simulink model "station_no_recovery"  (R2015a)
settings: Solver=ode45  StartTime=0  StopTime=5000  FixedStep=10  MaxStep=1  RelTol=1e-3
(part 1 of 4)
settings Model: Creator=Tzimisce  LastModifiedBy=Tzimisce
settings DebuggingCC: AlgebraicLoopMsg=none  ArtificialAlgebraicLoopMsg=none  InheritedTsInSrcMsg=none

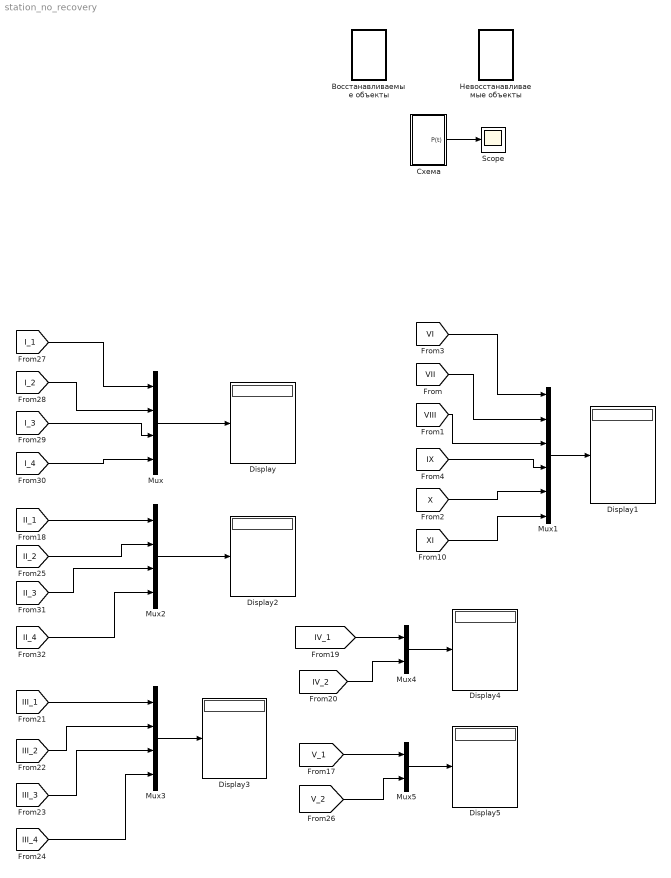
== system station_no_recovery ==
  Display{,1..5} (6 alike) : Display
  Mux : Mux
  Mux1 : Mux  Inputs=6
  Mux2 : Mux
  Mux3 : Mux
  Mux4 : Mux  Inputs=2
  Mux5 : Mux  Inputs=2
  Scope : Scope
      settings: TimeRange=5000
  Восстанавливаемые объекты : Subsystem  mask{lambda_exp1=0.0008664, lambda_norm1=100, M1=800, dp1=0.005, trec_1=5000, Pz1=0, dt1=10000, t_start1_1=0, t_start1_2=50, t_start1_3=100, t_start1_4=200, lambda_exp2=0.0002888, lambda_norm2=300, M2=2400, dp2=0.005, Pz2=0, dt2=10000, t_start2_1=50, t_start2_2=120, t_start2_3=310, t_start2_4=200, lambda_exp3=0.0002888, M3=2400, lambda_norm3=300, dp3=0.005, Pz3=0, dt3=10000, t_start3_1=50, t_start3_2=300, t_start3_3=1000, t_start3_4=150, lambda_exp4=0.0001733, lambda_norm4=500, M4=4000, dp4=0.005, Pz4=0, dt4=10000, t_start4_1=20, t_start4_2=220, lambda_exp5=0.0001733, lambda_norm5=500, M5=4000, dp5=0.005, Pz5=0, dt5=10000, t_start5_1=0, t_start5_2=500, trec_2=8000}
      mask prompts: lambda_exp1 "Параметр экспоненциального распределения ПАЭС"; lambda_norm1 "Параметр нормального распределения ПАЭС"; M1 "Мат ожидание нормального распределения ПАЭС"; dp1 "Доля деградации объекта ПАЭС"; trec_1 "Время капитального ремонта 1"; Pz1 "Заданная вероятность ПАЭС"; dt1 "Время восстановления ПАЭС"; t_start1_1 "Начальная наработка ПАЭС 1"; t_start1_2 "Начальная наработка ПАЭС 2"; t_start1_3 "Начальная наработка ПАЭС 3"; t_start1_4 "Начальная наработка ПАЭС 4"; lambda_exp2 "Параметр экспоненциального распределения УРАЛ"; lambda_norm2 "Параметр нормального распределения УРАЛ"; M2 "Мат ожидание нормального распределения УРАЛ"; dp2 "Доля деградации объекта УРАЛ"; Pz2 "Заданная вероятность УРАЛ"; dt2 "Время восстановления УРАЛ"; t_start2_1 "Начальная наработка УРАЛ 1"; t_start2_2 "Начальная наработка УРАЛ 2"; t_start2_3 "Начальная наработка УРАЛ 3"; t_start2_4 "Начальная наработка УРАЛ 4"; lambda_exp3 "Параметр экспоненциального распределения САТУРН"; M3 "Мат ожидание нормального распределения САТУРН"; lambda_norm3 "Параметр нормального распределения САТУРН"; dp3 "Доля деградации объекта САТУРН"; Pz3 "Заданная вероятность САТУРН"; dt3 "Время восстановления САТУРН"; t_start3_1 "Начальная наработка САТУРН 1"; t_start3_2 "Начальная наработка САТУРН 2"; t_start3_3 "Начальная наработка САТУРН 3"; t_start3_4 "Начальная наработка САТУРН 4"; lambda_exp4 "Параметр экспоненциального распределения ГТЭ"; lambda_norm4 "Параметр нормального распределения ГТЭ"; M4 "Мат ожидание нормального распределения ГТЭ"; dp4 "Доля деградации объекта ГТЭ"; Pz4 "Заданная вероятность ГТЭ"; dt4 "Время восстановления ГТЭ"; t_start4_1 "Начальная наработка ГТЭ 1"; t_start4_2 "Начальная наработка ГТЭ 2"; lambda_exp5 "Параметр экспоненциального распределения ЭГ"; lambda_norm5 "Параметр нормального распределения ЭГ"; M5 "Мат ожидание нормального распределения ЭГ"; dp5 "Доля деградации объекта ЭГ"; Pz5 "Заданная вероятность ЭГ"; dt5 "Время восстановления ЭГ"; t_start5_1 "Начальная наработка ЭГ 1"; t_start5_2 "Начальная наработка ЭГ 2"; trec_2 "Время капитального ремонта 2"
      mask DialogControl paes_container Prompt: ПАЭС
      mask DialogControl ural_container Prompt: УРАЛ
      mask DialogControl saturn_container Prompt: САТУРН
      mask DialogControl gte_container Prompt: ГТЭ
      mask DialogControl eg_container Prompt: ЭГ
  Невосстанавливаемые объекты : Subsystem  mask{lambda1=0.000024, lambda2=0.000001, lambda3=0.0000024, lambda4=0.000072, lambda5=0.000048}
      mask prompts: lambda1 "Параметр экспоненциального распределения ЗРУ (6кВт)"; lambda2 "Параметр экспоненциального распределения ВЩ"; lambda3 "Параметр экспоненциального распределения ГРУ"; lambda4 "Параметр экспоненциального распределения ТП"; lambda5 "Параметр экспоненциального распределения ЗРУ (35кВт)"
  Схема : Subsystem
  wires:
  Схема/1(P(t)) -> Scope/1
  Mux/1 -> Display/1
  [I_1] -> Mux/1
  [I_3] -> Mux/3
  [I_4] -> Mux/4
  [VI] -> Mux1/1
  [VII] -> Mux1/2
  [VIII] -> Mux1/3
  [IX] -> Mux1/4
  [X] -> Mux1/5
  [XI] -> Mux1/6
  Mux1/1 -> Display1/1
  [II_1] -> Mux2/1
  [III_1] -> Mux3/1
  [IV_1] -> Mux4/1
  [II_2] -> Mux2/2
  [III_2] -> Mux3/2
  [IV_2] -> Mux4/2
  [III_3] -> Mux3/3
  [III_4] -> Mux3/4
  [V_2] -> Mux5/2
  [I_2] -> Mux/2
  Mux2/1 -> Display2/1
  [II_3] -> Mux2/3
  [II_4] -> Mux2/4
  Mux3/1 -> Display3/1
  [V_1] -> Mux5/1
  Mux4/1 -> Display4/1
  Mux5/1 -> Display5/1

== system station_no_recovery/Восстанавливаемые объекты ==
  Constant : Constant  Value=trec_1
  Constant6 : Constant  Value=trec_2
  ГТЭ-6/6,3 : Subsystem
  ПАЭС-2500 : Subsystem
  САТУРН : Subsystem
  УРАЛ-6000 : Subsystem
  ЭГ-12 : Subsystem
  tag scope: trec1=global, trec2=global
  wires:
  Constant/1 -> [trec1]
  Constant6/1 -> [trec2]

== system station_no_recovery/Невосстанавливаемые объекты ==
  Constant : Constant
  Constant1 : Constant  Value=lambda4
  Constant2 : Constant  Value=lambda2
  Constant3 : Constant  Value=lambda3
  Constant4 : Constant  Value=lambda5
  Constant6 : Constant  Value=lambda1
  Element Exponential : Subsystem  mask(Element Exponential){}
      mask help:
      | <p>Возвращает вероятность безотказной работы невосстанавливаемого элемента
      | по экспоненциальному закону распределения.</p>
      | <p>Экспоненциальное (или показательное) распределение — абсолютно непрерывное
      | распределение, моделирующее время между двумя последовательными свершениями
      | одного и того же события.</p>
      | <p>Экспоненциальное распределение используют при оценке надежности сложных
      | технических систем, не подверженных износу и старению и в случаях, когда
      | отказы объектов имеют случайный характер.</p>
      mask Help:
      | <p>Возвращает вероятность безотказной работы невосстанавливаемого элемента по экспоненциальному
      | закону распределения.</p>
      | <p>Экспоненциальное распределение используют при оценке надежности сложных
      | технических систем, не подверженных износу и старению и в случаях, когда
      | отказы объектов имеют случайный характер.</p>
      | <p>Входной параметр λ - интенсивность событий в рассматриваемом потоке.</p>
      | <p>Выходной параметр P(t) - вероятность безотказной работы элемента.</p>
      mask Display:
      | image('images/png/exp.png')
      | port_label('input', 1, 'λ')
      | port_label('output', 1, 'P(t)')
  Element Exponential1 : Subsystem  mask(Element Exponential){}
      mask help:
      | <p>Возвращает вероятность безотказной работы невосстанавливаемого элемента
      | по экспоненциальному закону распределения.</p>
      | <p>Экспоненциальное (или показательное) распределение — абсолютно непрерывное
      | распределение, моделирующее время между двумя последовательными свершениями
      | одного и того же события.</p>
      | <p>Экспоненциальное распределение используют при оценке надежности сложных
      | технических систем, не подверженных износу и старению и в случаях, когда
      | отказы объектов имеют случайный характер.</p>
      mask Help:
      | <p>Возвращает вероятность безотказной работы невосстанавливаемого элемента по экспоненциальному
      | закону распределения.</p>
      | <p>Экспоненциальное распределение используют при оценке надежности сложных
      | технических систем, не подверженных износу и старению и в случаях, когда
      | отказы объектов имеют случайный характер.</p>
      | <p>Входной параметр λ - интенсивность событий в рассматриваемом потоке.</p>
      | <p>Выходной параметр P(t) - вероятность безотказной работы элемента.</p>
      mask Display:
      | image('images/png/exp.png')
      | port_label('input', 1, 'λ')
      | port_label('output', 1, 'P(t)')
  Element Exponential2 : Subsystem  mask(Element Exponential){}
      mask help:
      | <p>Возвращает вероятность безотказной работы невосстанавливаемого элемента
      | по экспоненциальному закону распределения.</p>
      | <p>Экспоненциальное (или показательное) распределение — абсолютно непрерывное
      | распределение, моделирующее время между двумя последовательными свершениями
      | одного и того же события.</p>
      | <p>Экспоненциальное распределение используют при оценке надежности сложных
      | технических систем, не подверженных износу и старению и в случаях, когда
      | отказы объектов имеют случайный характер.</p>
      mask Help:
      | <p>Возвращает вероятность безотказной работы невосстанавливаемого элемента по экспоненциальному
      | закону распределения.</p>
      | <p>Экспоненциальное распределение используют при оценке надежности сложных
      | технических систем, не подверженных износу и старению и в случаях, когда
      | отказы объектов имеют случайный характер.</p>
      | <p>Входной параметр λ - интенсивность событий в рассматриваемом потоке.</p>
      | <p>Выходной параметр P(t) - вероятность безотказной работы элемента.</p>
      mask Display:
      | image('images/png/exp.png')
      | port_label('input', 1, 'λ')
      | port_label('output', 1, 'P(t)')
  Element Exponential3 : Subsystem  mask(Element Exponential){}
      mask help:
      | <p>Возвращает вероятность безотказной работы невосстанавливаемого элемента
      | по экспоненциальному закону распределения.</p>
      | <p>Экспоненциальное (или показательное) распределение — абсолютно непрерывное
      | распределение, моделирующее время между двумя последовательными свершениями
      | одного и того же события.</p>
      | <p>Экспоненциальное распределение используют при оценке надежности сложных
      | технических систем, не подверженных износу и старению и в случаях, когда
      | отказы объектов имеют случайный характер.</p>
      mask Help:
      | <p>Возвращает вероятность безотказной работы невосстанавливаемого элемента по экспоненциальному
      | закону распределения.</p>
      | <p>Экспоненциальное распределение используют при оценке надежности сложных
      | технических систем, не подверженных износу и старению и в случаях, когда
      | отказы объектов имеют случайный характер.</p>
      | <p>Входной параметр λ - интенсивность событий в рассматриваемом потоке.</p>
      | <p>Выходной параметр P(t) - вероятность безотказной работы элемента.</p>
      mask Display:
      | image('images/png/exp.png')
      | port_label('input', 1, 'λ')
      | port_label('output', 1, 'P(t)')
  Element Exponential4 : Subsystem  mask(Element Exponential){}
      mask help:
      | <p>Возвращает вероятность безотказной работы невосстанавливаемого элемента
      | по экспоненциальному закону распределения.</p>
      | <p>Экспоненциальное (или показательное) распределение — абсолютно непрерывное
      | распределение, моделирующее время между двумя последовательными свершениями
      | одного и того же события.</p>
      | <p>Экспоненциальное распределение используют при оценке надежности сложных
      | технических систем, не подверженных износу и старению и в случаях, когда
      | отказы объектов имеют случайный характер.</p>
      mask Help:
      | <p>Возвращает вероятность безотказной работы невосстанавливаемого элемента по экспоненциальному
      | закону распределения.</p>
      | <p>Экспоненциальное распределение используют при оценке надежности сложных
      | технических систем, не подверженных износу и старению и в случаях, когда
      | отказы объектов имеют случайный характер.</p>
      | <p>Входной параметр λ - интенсивность событий в рассматриваемом потоке.</p>
      | <p>Выходной параметр P(t) - вероятность безотказной работы элемента.</p>
      mask Display:
      | image('images/png/exp.png')
      | port_label('input', 1, 'λ')
      | port_label('output', 1, 'P(t)')
  tag scope: IX=global, VI=global, VII=global, VIII=global, X=global, XI=global
  wires:
  Constant1/1 -> Element Exponential3/1("lambda ")
  Element Exponential/1(P(t)1) -> [VI]
  Constant/1 -> [XI]
  Constant3/1 -> Element Exponential2/1("lambda ")
  Element Exponential3/1(P(t)1) -> [IX]
  Constant4/1 -> Element Exponential4/1("lambda ")
  Constant2/1 -> Element Exponential1/1("lambda ")
  Element Exponential4/1(P(t)1) -> [X]
  Element Exponential1/1(P(t)1) -> [VII]
  Element Exponential2/1(P(t)1) -> [VIII]
  Constant6/1 -> Element Exponential/1("lambda ")

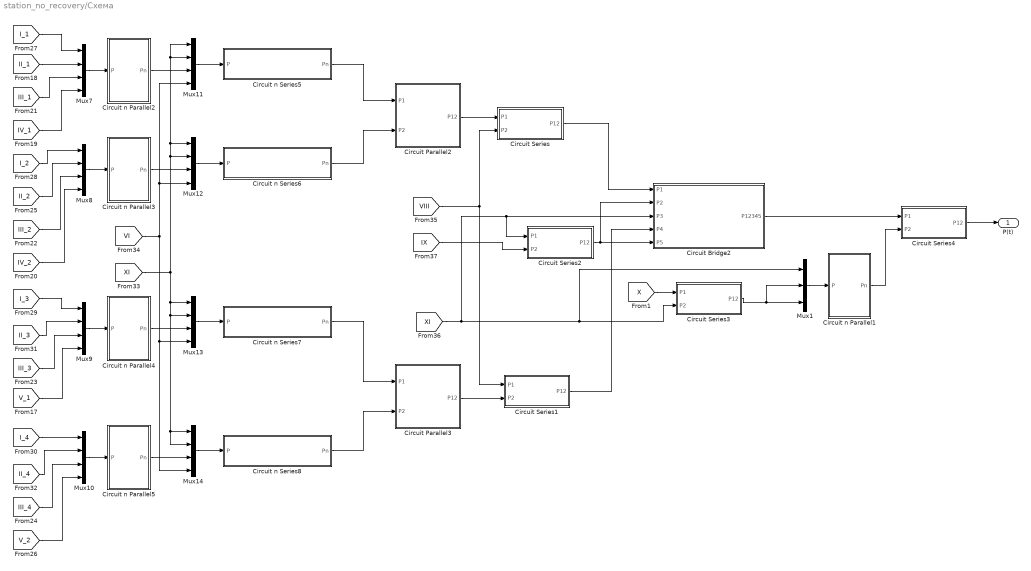
== system station_no_recovery/Схема ==
  Mux1 : Mux  Inputs=3
  Mux{7..14} (8 alike) : Mux
  Сircuit Bridge2 : Subsystem  mask(Сircuit Bridge){}
      mask help:
      | <p>Возвращает вероятность безотказной работы пяти элементов, соединенных
      | мостиковой схемой.</p>
      | <p>Мостиковой схемой называется параллельное соединение последовательных
      | цепочек элементов с диагональными элементами, включенными между узлами
      | различных параллельных ветвей.</p>
      | <p>Работоспособность мостиковой схемы зависит не только от количества отказавших
      | элементов, но и от их положения в структурной схеме.</p>
      mask Help:
      | <p>Возвращает вероятность безотказной работы пяти элементов, соединенных
      | мостиковой схемой.</p>
      | <p>Работоспособность мостиковой схемы зависит не только от количества отказавших
      | элементов, но и от их положения в структурной схеме. При одновременном отказе
      | элементов 1 и 4, или 2 и 5, или 2, 3 и 4 и т.д. схема окажется неработоспособной.
      | Но отказ элементов 1 и 5, или 2 и 4, или 1, 3 и 4, или 2, 3 и 5 к отказу
      | системы не приводит.</p>
      | <p>Входные параметры:</p>
      | <p>P1 - вероятность безотказной работы первого элемента,</p>
      | <p>P2 - вероятность безотказной работы второго элемента,</p>
      | <p>P3 - вероятность безотказной работы третьего элемента,</p>
      | <p>P4 - вероятность безотказной работы четвертого элемента,</p>
      | <p>P5 - вероятность безотказной работы пятого элемента.</p>
      | <p>Выходной параметр P(t) - вероятность безотказной работы всех элементов.</p>
      mask Display:
      | image('images\png\bridge.png')
      | port_label('input', 1, 'P1')
      | port_label('input', 2, 'P2')
      | port_label('input', 3, 'P3')
      | port_label('input', 4, 'P4')
      | port_label('input', 5, 'P5')
      | port_label('output', 1, 'P')
  Сircuit Parallel2 : Subsystem  mask(Сircuit Parallel){}
      mask help:
      | <p>Возвращает вероятность безотказной работы двух параллельно соединенных
      | элементов.</p>
      | <p>В системе с параллельной структурой отказ системы в целом происходит только
      | при отказе всех элементов.</p>
      mask Help:
      | <p>Возвращает вероятность безотказной работы двух параллельно соединенных
      | элементов.</p>
      | <p>Входные параметры:</p>
      | <p>P1 - вероятность безотказной работы первого элемента,</p>
      | <p>P2 - вероятность безотказной работы второго элемента.</p>
      | <p>Выходной параметр P12 - вероятность безотказной работы двух параллельно
      | соединенных элементов.</p>
      mask Display:
      | image('images/png/parallel2.png')
      | port_label('input', 1, 'P1')
      | port_label('input', 2, 'P2')
      | port_label('output', 1, 'P12')
  Сircuit Parallel3 : Subsystem  mask(Сircuit Parallel){}
      mask help:
      | <p>Возвращает вероятность безотказной работы двух параллельно соединенных
      | элементов.</p>
      | <p>В системе с параллельной структурой отказ системы в целом происходит только
      | при отказе всех элементов.</p>
      mask Help:
      | <p>Возвращает вероятность безотказной работы двух параллельно соединенных
      | элементов.</p>
      | <p>Входные параметры:</p>
      | <p>P1 - вероятность безотказной работы первого элемента,</p>
      | <p>P2 - вероятность безотказной работы второго элемента.</p>
      | <p>Выходной параметр P12 - вероятность безотказной работы двух параллельно
      | соединенных элементов.</p>
      mask Display:
      | image('images/png/parallel2.png')
      | port_label('input', 1, 'P1')
      | port_label('input', 2, 'P2')
      | port_label('output', 1, 'P12')
  Сircuit Series : Subsystem  mask(Сircuit Series){}
      mask help:
      | <p>Возвращает вероятность безотказной работы двух последовательно соединенных
      | элементов.</p>
      | <p>В системе с последовательной структурой отказ любого компонента приводит
      | к отказу системы в целом.</p>
      mask Help:
      | <p>Возвращает вероятность безотказной работы двух последовательно соединенных
      | элементов.</p>
      | <p>Входные параметры:</p>
      | <p>P1 - вероятность безотказной работы первого элемента,</p>
      | <p>P2 - вероятность безотказной работы второго элемента.</p>
      | <p>Выходной параметр P12 - вероятность безотказной работы двух последовательно
      | соединенных элементов.</p>
      mask Display:
      | image('images/png/series2.png')
      | port_label('input', 1, 'P1')
      | port_label('input', 2, 'P2')
      | port_label('output', 1, 'P12')
  Сircuit Series1 : Subsystem  mask(Сircuit Series){}
      mask help:
      | <p>Возвращает вероятность безотказной работы двух последовательно соединенных
      | элементов.</p>
      | <p>В системе с последовательной структурой отказ любого компонента приводит
      | к отказу системы в целом.</p>
      mask Help:
      | <p>Возвращает вероятность безотказной работы двух последовательно соединенных
      | элементов.</p>
      | <p>Входные параметры:</p>
      | <p>P1 - вероятность безотказной работы первого элемента,</p>
      | <p>P2 - вероятность безотказной работы второго элемента.</p>
      | <p>Выходной параметр P12 - вероятность безотказной работы двух последовательно
      | соединенных элементов.</p>
      mask Display:
      | image('images/png/series2.png')
      | port_label('input', 1, 'P1')
      | port_label('input', 2, 'P2')
      | port_label('output', 1, 'P12')
  Сircuit Series2 : Subsystem  mask(Сircuit Series){}
      mask help:
      | <p>Возвращает вероятность безотказной работы двух последовательно соединенных
      | элементов.</p>
      | <p>В системе с последовательной структурой отказ любого компонента приводит
      | к отказу системы в целом.</p>
      mask Help:
      | <p>Возвращает вероятность безотказной работы двух последовательно соединенных
      | элементов.</p>
      | <p>Входные параметры:</p>
      | <p>P1 - вероятность безотказной работы первого элемента,</p>
      | <p>P2 - вероятность безотказной работы второго элемента.</p>
      | <p>Выходной параметр P12 - вероятность безотказной работы двух последовательно
      | соединенных элементов.</p>
      mask Display:
      | image('images/png/series2.png')
      | port_label('input', 1, 'P1')
      | port_label('input', 2, 'P2')
      | port_label('output', 1, 'P12')
  Сircuit Series3 : Subsystem  mask(Сircuit Series){}
      mask help:
      | <p>Возвращает вероятность безотказной работы двух последовательно соединенных
      | элементов.</p>
      | <p>В системе с последовательной структурой отказ любого компонента приводит
      | к отказу системы в целом.</p>
      mask Help:
      | <p>Возвращает вероятность безотказной работы двух последовательно соединенных
      | элементов.</p>
      | <p>Входные параметры:</p>
      | <p>P1 - вероятность безотказной работы первого элемента,</p>
      | <p>P2 - вероятность безотказной работы второго элемента.</p>
      | <p>Выходной параметр P12 - вероятность безотказной работы двух последовательно
      | соединенных элементов.</p>
      mask Display:
      | image('images/png/series2.png')
      | port_label('input', 1, 'P1')
      | port_label('input', 2, 'P2')
      | port_label('output', 1, 'P12')
  Сircuit Series4 : Subsystem  mask(Сircuit Series){}
      mask help:
      | <p>Возвращает вероятность безотказной работы двух последовательно соединенных
      | элементов.</p>
      | <p>В системе с последовательной структурой отказ любого компонента приводит
      | к отказу системы в целом.</p>
      mask Help:
      | <p>Возвращает вероятность безотказной работы двух последовательно соединенных
      | элементов.</p>
      | <p>Входные параметры:</p>
      | <p>P1 - вероятность безотказной работы первого элемента,</p>
      | <p>P2 - вероятность безотказной работы второго элемента.</p>
      | <p>Выходной параметр P12 - вероятность безотказной работы двух последовательно
      | соединенных элементов.</p>
      mask Display:
      | image('images/png/series2.png')
      | port_label('input', 1, 'P1')
      | port_label('input', 2, 'P2')
      | port_label('output', 1, 'P12')
  Сircuit n Parallel1 : Subsystem  mask(Сircuit n Parallel){}
      mask help:
      | <p>Возвращает вероятность безотказной работы n параллельно соединенных
      | элементов.</p>
      | <p>В системе с параллельной структурой отказ системы в целом происходит только
      | при отказе всех элементов.</p>
      mask Help:
      | <p>Возвращает вероятность безотказной работы n параллельно соединенных
      | элементов.</p>
      | <p>Входной параметр P - массив вероятностей безотказной работы элементов.</p>
      | <p>Выходной параметр Pт - вероятность безотказной работы n параллельно
      | соединенных элементов.</p>
      mask Display:
      | image('images\png\parallel.png')
      | port_label('input', 1, 'P')
      | port_label('output', 1, 'Pn')
  Сircuit n Parallel2 : Subsystem  mask(Сircuit n Parallel){}
      mask help:
      | <p>Возвращает вероятность безотказной работы n параллельно соединенных
      | элементов.</p>
      | <p>В системе с параллельной структурой отказ системы в целом происходит только
      | при отказе всех элементов.</p>
      mask Help:
      | <p>Возвращает вероятность безотказной работы n параллельно соединенных
      | элементов.</p>
      | <p>Входной параметр P - массив вероятностей безотказной работы элементов.</p>
      | <p>Выходной параметр Pт - вероятность безотказной работы n параллельно
      | соединенных элементов.</p>
      mask Display:
      | image('images\png\parallel.png')
      | port_label('input', 1, 'P')
      | port_label('output', 1, 'Pn')
  Сircuit n Parallel3 : Subsystem  mask(Сircuit n Parallel){}
      mask help:
      | <p>Возвращает вероятность безотказной работы n параллельно соединенных
      | элементов.</p>
      | <p>В системе с параллельной структурой отказ системы в целом происходит только
      | при отказе всех элементов.</p>
      mask Help:
      | <p>Возвращает вероятность безотказной работы n параллельно соединенных
      | элементов.</p>
      | <p>Входной параметр P - массив вероятностей безотказной работы элементов.</p>
      | <p>Выходной параметр Pт - вероятность безотказной работы n параллельно
      | соединенных элементов.</p>
      mask Display:
      | image('images\png\parallel.png')
      | port_label('input', 1, 'P')
      | port_label('output', 1, 'Pn')
  Сircuit n Parallel4 : Subsystem  mask(Сircuit n Parallel){}
      mask help:
      | <p>Возвращает вероятность безотказной работы n параллельно соединенных
      | элементов.</p>
      | <p>В системе с параллельной структурой отказ системы в целом происходит только
      | при отказе всех элементов.</p>
      mask Help:
      | <p>Возвращает вероятность безотказной работы n параллельно соединенных
      | элементов.</p>
      | <p>Входной параметр P - массив вероятностей безотказной работы элементов.</p>
      | <p>Выходной параметр Pт - вероятность безотказной работы n параллельно
      | соединенных элементов.</p>
      mask Display:
      | image('images\png\parallel.png')
      | port_label('input', 1, 'P')
      | port_label('output', 1, 'Pn')
  Сircuit n Parallel5 : Subsystem  mask(Сircuit n Parallel){}
      mask help:
      | <p>Возвращает вероятность безотказной работы n параллельно соединенных
      | элементов.</p>
      | <p>В системе с параллельной структурой отказ системы в целом происходит только
      | при отказе всех элементов.</p>
      mask Help:
      | <p>Возвращает вероятность безотказной работы n параллельно соединенных
      | элементов.</p>
      | <p>Входной параметр P - массив вероятностей безотказной работы элементов.</p>
      | <p>Выходной параметр Pт - вероятность безотказной работы n параллельно
      | соединенных элементов.</p>
      mask Display:
      | image('images\png\parallel.png')
      | port_label('input', 1, 'P')
      | port_label('output', 1, 'Pn')
  Сircuit n Series5 : Subsystem  mask(Сircuit n Series){}
      mask help:
      | <p>Возвращает вероятность безотказной работы n последовательно соединенных
      | элементов.</p>
      | <p>В системе с последовательной структурой отказ любого компонента приводит
      | к отказу системы в целом.</p>
      mask Help:
      | <p>Возвращает вероятность безотказной работы n последовательно соединенных
      | элементов.</p>
      | <p>Входной параметр P - массив вероятностей безотказной работы n элементов.</p>
      | <p>Выходной параметр Pn - вероятность безотказной работы n последовательно
      | соединенных элементов.</p>
      mask Display:
      | image('images\png\series.png')
      | port_label('input', 1, 'P')
      | port_label('output', 1, 'Pn')
  Сircuit n Series6 : Subsystem  mask(Сircuit n Series){}
      mask help:
      | <p>Возвращает вероятность безотказной работы n последовательно соединенных
      | элементов.</p>
      | <p>В системе с последовательной структурой отказ любого компонента приводит
      | к отказу системы в целом.</p>
      mask Help:
      | <p>Возвращает вероятность безотказной работы n последовательно соединенных
      | элементов.</p>
      | <p>Входной параметр P - массив вероятностей безотказной работы n элементов.</p>
      | <p>Выходной параметр Pn - вероятность безотказной работы n последовательно
      | соединенных элементов.</p>
      mask Display:
      | image('images\png\series.png')
      | port_label('input', 1, 'P')
      | port_label('output', 1, 'Pn')
  Сircuit n Series7 : Subsystem  mask(Сircuit n Series){}
      mask help:
      | <p>Возвращает вероятность безотказной работы n последовательно соединенных
      | элементов.</p>
      | <p>В системе с последовательной структурой отказ любого компонента приводит
      | к отказу системы в целом.</p>
      mask Help:
      | <p>Возвращает вероятность безотказной работы n последовательно соединенных
      | элементов.</p>
      | <p>Входной параметр P - массив вероятностей безотказной работы n элементов.</p>
      | <p>Выходной параметр Pn - вероятность безотказной работы n последовательно
      | соединенных элементов.</p>
      mask Display:
      | image('images\png\series.png')
      | port_label('input', 1, 'P')
      | port_label('output', 1, 'Pn')
  Сircuit n Series8 : Subsystem  mask(Сircuit n Series){}
      mask help:
      | <p>Возвращает вероятность безотказной работы n последовательно соединенных
      | элементов.</p>
      | <p>В системе с последовательной структурой отказ любого компонента приводит
      | к отказу системы в целом.</p>
      mask Help:
      | <p>Возвращает вероятность безотказной работы n последовательно соединенных
      | элементов.</p>
      | <p>Входной параметр P - массив вероятностей безотказной работы n элементов.</p>
      | <p>Выходной параметр Pn - вероятность безотказной работы n последовательно
      | соединенных элементов.</p>
      mask Display:
      | image('images\png\series.png')
      | port_label('input', 1, 'P')
      | port_label('output', 1, 'Pn')
  P(t) : Outport
  wires:
  [I_1] -> Mux7/1
  [II_1] -> Mux7/2
  [III_1] -> Mux7/3
  [IV_1] -> Mux7/4
  [I_2] -> Mux8/1
  [II_2] -> Mux8/2
  [III_2] -> Mux8/3
  [IV_2] -> Mux8/4
  [I_3] -> Mux9/1
  [II_3] -> Mux9/2
  [III_3] -> Mux9/3
  [V_1] -> Mux9/4
  [I_4] -> Mux10/1
  [II_4] -> Mux10/2
  [III_4] -> Mux10/3
  [V_2] -> Mux10/4
  Mux7/1 -> Сircuit n Parallel2/1(P)
  Mux8/1 -> Сircuit n Parallel3/1(P)
  Mux9/1 -> Сircuit n Parallel4/1(P)
  Mux10/1 -> Сircuit n Parallel5/1(P)
  Сircuit n Parallel2/1(Pn) -> Mux11/3
  Сircuit n Parallel3/1(Pn) -> Mux12/3
  Сircuit n Parallel4/1(Pn) -> Mux13/3
  Сircuit n Parallel5/1(Pn) -> Mux14/3
  [XI] -> Mux12/2, Mux12/1, Mux11/2, Mux11/1, Mux14/2, Mux14/1, Mux13/2, Mux13/1
  [VI] -> Mux14/4, Mux13/4, Mux11/4, Mux12/4
  Mux11/1 -> Сircuit n Series5/1(P)
  Сircuit n Series5/1(Pn) -> Сircuit Parallel2/1(P1)
  Mux12/1 -> Сircuit n Series6/1(P)
  Сircuit n Series6/1(Pn) -> Сircuit Parallel2/2(P2)
  Mux13/1 -> Сircuit n Series7/1(P)
  Сircuit n Series7/1(Pn) -> Сircuit Parallel3/1(P1)
  Mux14/1 -> Сircuit n Series8/1(P)
  Сircuit n Series8/1(Pn) -> Сircuit Parallel3/2(P2)
  Сircuit Series4/1(P12) -> P(t)/1
  Сircuit Parallel2/1(P12) -> Сircuit Series/1(P1)
  [VIII] -> Сircuit Series/2(P2), Сircuit Series1/1(P1)
  Сircuit Parallel3/1(P12) -> Сircuit Series1/2(P2)
  Сircuit Series/1(P12) -> Сircuit Bridge2/1(P1)
  Сircuit Series1/1(P12) -> Сircuit Bridge2/4(P4)
  [XI] -> Mux1/1, Сircuit Series3/2(P2), Сircuit Bridge2/3(P3), Сircuit Series2/1(P1)
  [IX] -> Сircuit Series2/2(P2)
  Сircuit Series2/1(P12) -> Сircuit Bridge2/2(P2), Сircuit Bridge2/5(P5)
  [X] -> Сircuit Series3/1(P1)
  Сircuit Series3/1(P12) -> Mux1/2, Mux1/3
  Mux1/1 -> Сircuit n Parallel1/1(P)
  Сircuit Bridge2/1(P12345) -> Сircuit Series4/1(P1)
  Сircuit n Parallel1/1(Pn) -> Сircuit Series4/2(P2)

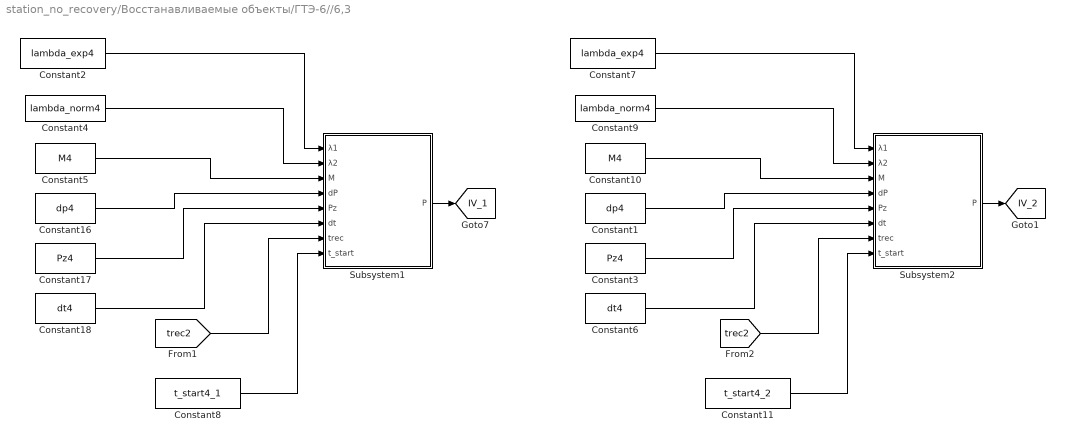
== system station_no_recovery/Восстанавливаемые объекты/ГТЭ-6//6,3 ==
  Constant1 : Constant  Value=dp4
  Constant10 : Constant  Value=M4
  Constant11 : Constant  Value=t_start4_2
  Constant16 : Constant  Value=dp4
  Constant17 : Constant  Value=Pz4
  Constant18 : Constant  Value=dt4
  Constant2 : Constant  Value=lambda_exp4
  Constant3 : Constant  Value=Pz4
  Constant4 : Constant  Value=lambda_norm4
  Constant5 : Constant  Value=M4
  Constant6 : Constant  Value=dt4
  Constant7 : Constant  Value=lambda_exp4
  Constant8 : Constant  Value=t_start4_1
  Constant9 : Constant  Value=lambda_norm4
  Subsystem1 : Subsystem
  Subsystem2 : Subsystem
  tag scope: IV_1=global, IV_2=global
  wires:
  Constant16/1 -> Subsystem1/4(dP)
  Constant18/1 -> Subsystem1/6(dt)
  Constant8/1 -> Subsystem1/8(t_start)
  Constant4/1 -> Subsystem1/2(λ2)
  Constant17/1 -> Subsystem1/5(Pz)
  Subsystem1/1(P) -> [IV_1]
  Constant2/1 -> Subsystem1/1(λ1)
  Constant5/1 -> Subsystem1/3(M)
  [trec2] -> Subsystem1/7(trec)
  Constant1/1 -> Subsystem2/4(dP)
  Constant6/1 -> Subsystem2/6(dt)
  Constant11/1 -> Subsystem2/8(t_start)
  Constant9/1 -> Subsystem2/2(λ2)
  Constant3/1 -> Subsystem2/5(Pz)
  Subsystem2/1(P) -> [IV_2]
  Constant7/1 -> Subsystem2/1(λ1)
  Constant10/1 -> Subsystem2/3(M)
  [trec2] -> Subsystem2/7(trec)

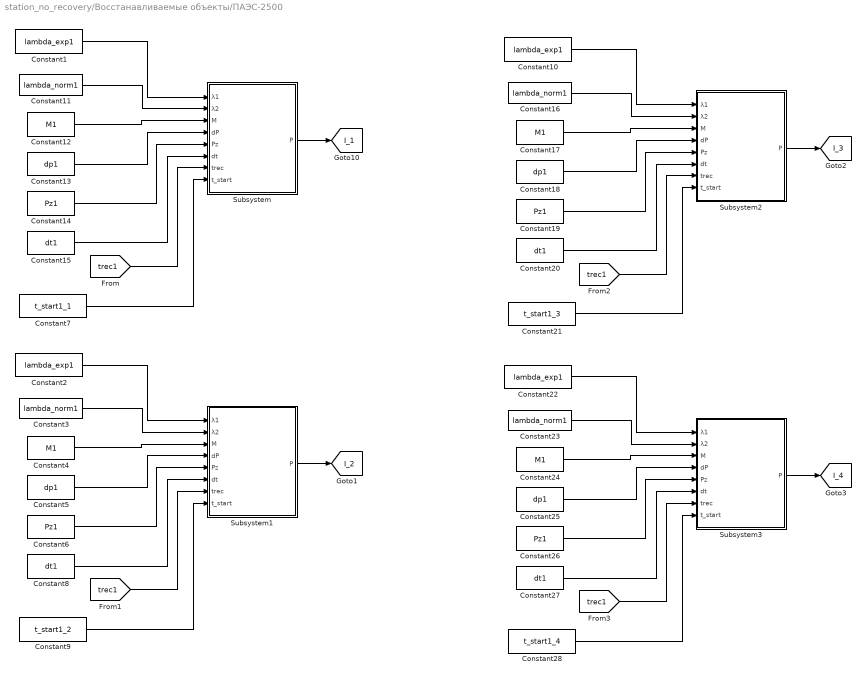
== system station_no_recovery/Восстанавливаемые объекты/ПАЭС-2500 ==
  Constant{1..2,10,22} (4 alike) : Constant  Value=lambda_exp1
  Constant{3,11,16,23} (4 alike) : Constant  Value=lambda_norm1
  Constant{4,12,17,24} (4 alike) : Constant  Value=M1
  Constant{5,13,18,25} (4 alike) : Constant  Value=dp1
  Constant{6,14,19,26} (4 alike) : Constant  Value=Pz1
  Constant{8,15,20,27} (4 alike) : Constant  Value=dt1
  Constant21 : Constant  Value=t_start1_3
  Constant28 : Constant  Value=t_start1_4
  Constant7 : Constant  Value=t_start1_1
  Constant9 : Constant  Value=t_start1_2
  Subsystem : Subsystem
  Subsystem1 : Subsystem
  Subsystem2 : Subsystem
  Subsystem3 : Subsystem
  tag scope: I_1=global, I_2=global, I_3=global, I_4=global
  wires:
  Constant11/1 -> Subsystem/2(λ2)
  Constant13/1 -> Subsystem/4(dP)
  Constant14/1 -> Subsystem/5(Pz)
  Constant12/1 -> Subsystem/3(M)
  Constant15/1 -> Subsystem/6(dt)
  Constant1/1 -> Subsystem/1(λ1)
  Constant7/1 -> Subsystem/8(t_start)
  [trec1] -> Subsystem/7(trec)
  Subsystem/1(P) -> [I_1]
  Constant3/1 -> Subsystem1/2(λ2)
  Constant5/1 -> Subsystem1/4(dP)
  Constant6/1 -> Subsystem1/5(Pz)
  Constant4/1 -> Subsystem1/3(M)
  Constant8/1 -> Subsystem1/6(dt)
  Constant2/1 -> Subsystem1/1(λ1)
  Constant9/1 -> Subsystem1/8(t_start)
  [trec1] -> Subsystem1/7(trec)
  Subsystem1/1(P) -> [I_2]
  Constant16/1 -> Subsystem2/2(λ2)
  Constant18/1 -> Subsystem2/4(dP)
  Constant19/1 -> Subsystem2/5(Pz)
  Constant17/1 -> Subsystem2/3(M)
  Constant20/1 -> Subsystem2/6(dt)
  Constant10/1 -> Subsystem2/1(λ1)
  Constant21/1 -> Subsystem2/8(t_start)
  [trec1] -> Subsystem2/7(trec)
  Subsystem2/1(P) -> [I_3]
  Constant23/1 -> Subsystem3/2(λ2)
  Constant25/1 -> Subsystem3/4(dP)
  Constant26/1 -> Subsystem3/5(Pz)
  Constant24/1 -> Subsystem3/3(M)
  Constant27/1 -> Subsystem3/6(dt)
  Constant22/1 -> Subsystem3/1(λ1)
  Constant28/1 -> Subsystem3/8(t_start)
  [trec1] -> Subsystem3/7(trec)
  Subsystem3/1(P) -> [I_4]

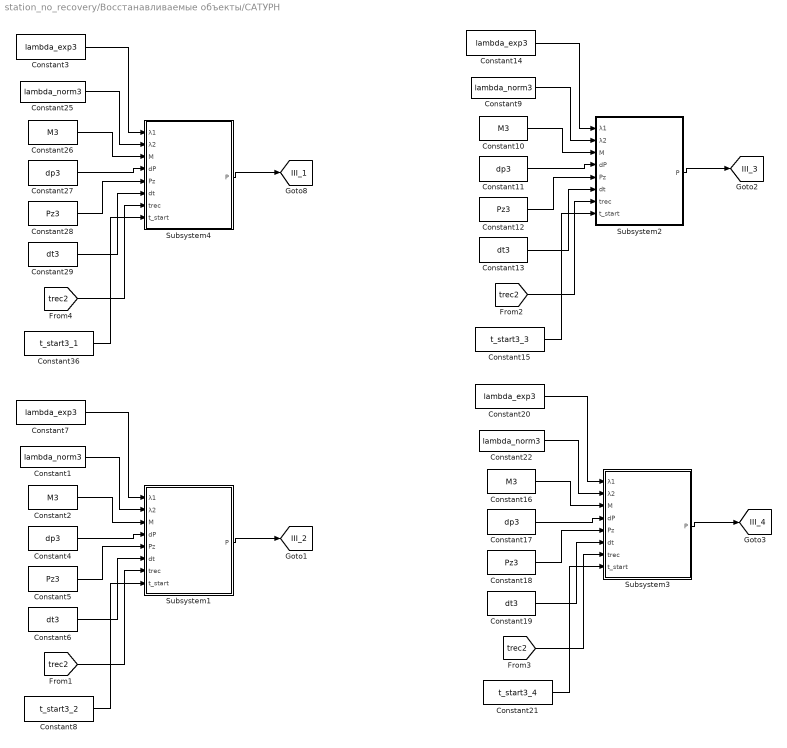
== system station_no_recovery/Восстанавливаемые объекты/САТУРН ==
  Constant{1,9,22,25} (4 alike) : Constant  Value=lambda_norm3
  Constant{2,10,16,26} (4 alike) : Constant  Value=M3
  Constant{4,11,17,27} (4 alike) : Constant  Value=dp3
  Constant{5,12,18,28} (4 alike) : Constant  Value=Pz3
  Constant{6,13,19,29} (4 alike) : Constant  Value=dt3
  Constant{3,7,14,20} (4 alike) : Constant  Value=lambda_exp3
  Constant15 : Constant  Value=t_start3_3
  Constant21 : Constant  Value=t_start3_4
  Constant36 : Constant  Value=t_start3_1
  Constant8 : Constant  Value=t_start3_2
  Subsystem1 : Subsystem
  Subsystem2 : Subsystem
  Subsystem3 : Subsystem
  Subsystem4 : Subsystem
  tag scope: III_1=global, III_2=global, III_3=global, III_4=global
  wires:
  Constant3/1 -> Subsystem4/1(λ1)
  Constant28/1 -> Subsystem4/5(Pz)
  Subsystem4/1(P) -> [III_1]
  Constant27/1 -> Subsystem4/4(dP)
  [trec2] -> Subsystem4/7(trec)
  Constant25/1 -> Subsystem4/2(λ2)
  Constant29/1 -> Subsystem4/6(dt)
  Constant26/1 -> Subsystem4/3(M)
  Constant36/1 -> Subsystem4/8(t_start)
  Constant7/1 -> Subsystem1/1(λ1)
  Constant5/1 -> Subsystem1/5(Pz)
  Subsystem1/1(P) -> [III_2]
  Constant4/1 -> Subsystem1/4(dP)
  [trec2] -> Subsystem1/7(trec)
  Constant1/1 -> Subsystem1/2(λ2)
  Constant6/1 -> Subsystem1/6(dt)
  Constant2/1 -> Subsystem1/3(M)
  Constant8/1 -> Subsystem1/8(t_start)
  Constant14/1 -> Subsystem2/1(λ1)
  Constant12/1 -> Subsystem2/5(Pz)
  Subsystem2/1(P) -> [III_3]
  Constant11/1 -> Subsystem2/4(dP)
  [trec2] -> Subsystem2/7(trec)
  Constant9/1 -> Subsystem2/2(λ2)
  Constant13/1 -> Subsystem2/6(dt)
  Constant10/1 -> Subsystem2/3(M)
  Constant15/1 -> Subsystem2/8(t_start)
  Constant20/1 -> Subsystem3/1(λ1)
  Constant18/1 -> Subsystem3/5(Pz)
  Subsystem3/1(P) -> [III_4]
  Constant17/1 -> Subsystem3/4(dP)
  [trec2] -> Subsystem3/7(trec)
  Constant22/1 -> Subsystem3/2(λ2)
  Constant19/1 -> Subsystem3/6(dt)
  Constant16/1 -> Subsystem3/3(M)
  Constant21/1 -> Subsystem3/8(t_start)

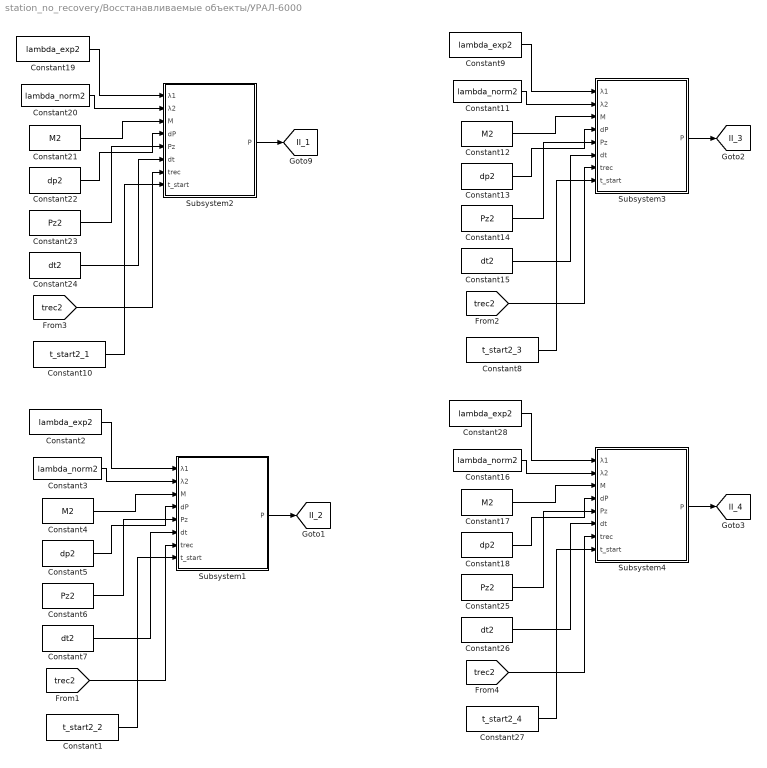
== system station_no_recovery/Восстанавливаемые объекты/УРАЛ-6000 ==
  Constant1 : Constant  Value=t_start2_2
  Constant10 : Constant  Value=t_start2_1
  Constant{3,11,16,20} (4 alike) : Constant  Value=lambda_norm2
  Constant{4,12,17,21} (4 alike) : Constant  Value=M2
  Constant{5,13,18,22} (4 alike) : Constant  Value=dp2
  Constant{6,14,23,25} (4 alike) : Constant  Value=Pz2
  Constant{7,15,24,26} (4 alike) : Constant  Value=dt2
  Constant{2,9,19,28} (4 alike) : Constant  Value=lambda_exp2
  Constant27 : Constant  Value=t_start2_4
  Constant8 : Constant  Value=t_start2_3
  Subsystem1 : Subsystem
  Subsystem2 : Subsystem
  Subsystem3 : Subsystem
  Subsystem4 : Subsystem
  tag scope: II_1=global, II_2=global, II_3=global, II_4=global
  wires:
  Constant23/1 -> Subsystem2/5(Pz)
  Constant19/1 -> Subsystem2/1(λ1)
  Constant22/1 -> Subsystem2/4(dP)
  Constant24/1 -> Subsystem2/6(dt)
  Constant21/1 -> Subsystem2/3(M)
  Constant20/1 -> Subsystem2/2(λ2)
  [trec2] -> Subsystem2/7(trec)
  Subsystem2/1(P) -> [II_1]
  Constant10/1 -> Subsystem2/8(t_start)
  Constant6/1 -> Subsystem1/5(Pz)
  Constant2/1 -> Subsystem1/1(λ1)
  Constant5/1 -> Subsystem1/4(dP)
  Constant7/1 -> Subsystem1/6(dt)
  Constant4/1 -> Subsystem1/3(M)
  Constant3/1 -> Subsystem1/2(λ2)
  [trec2] -> Subsystem1/7(trec)
  Subsystem1/1(P) -> [II_2]
  Constant1/1 -> Subsystem1/8(t_start)
  Constant14/1 -> Subsystem3/5(Pz)
  Constant9/1 -> Subsystem3/1(λ1)
  Constant13/1 -> Subsystem3/4(dP)
  Constant15/1 -> Subsystem3/6(dt)
  Constant12/1 -> Subsystem3/3(M)
  Constant11/1 -> Subsystem3/2(λ2)
  [trec2] -> Subsystem3/7(trec)
  Subsystem3/1(P) -> [II_3]
  Constant8/1 -> Subsystem3/8(t_start)
  Constant25/1 -> Subsystem4/5(Pz)
  Constant28/1 -> Subsystem4/1(λ1)
  Constant18/1 -> Subsystem4/4(dP)
  Constant26/1 -> Subsystem4/6(dt)
  Constant17/1 -> Subsystem4/3(M)
  Constant16/1 -> Subsystem4/2(λ2)
  [trec2] -> Subsystem4/7(trec)
  Subsystem4/1(P) -> [II_4]
  Constant27/1 -> Subsystem4/8(t_start)

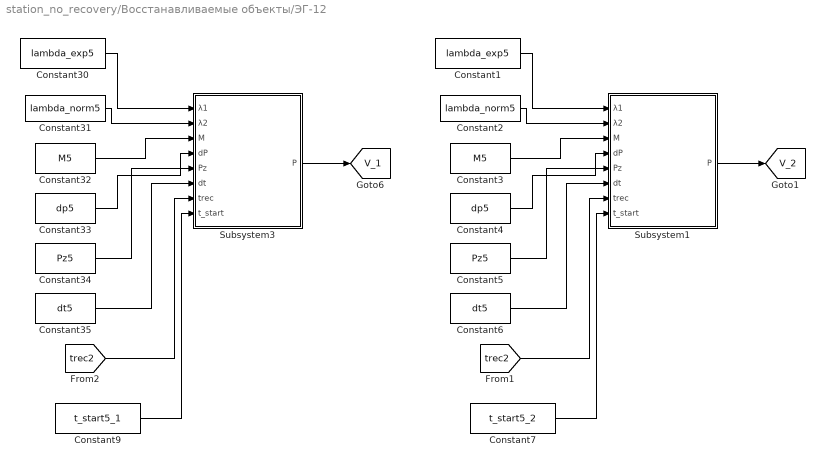
== system station_no_recovery/Восстанавливаемые объекты/ЭГ-12 ==
  Constant1 : Constant  Value=lambda_exp5
  Constant2 : Constant  Value=lambda_norm5
  Constant3 : Constant  Value=M5
  Constant30 : Constant  Value=lambda_exp5
  Constant31 : Constant  Value=lambda_norm5
  Constant32 : Constant  Value=M5
  Constant33 : Constant  Value=dp5
  Constant34 : Constant  Value=Pz5
  Constant35 : Constant  Value=dt5
  Constant4 : Constant  Value=dp5
  Constant5 : Constant  Value=Pz5
  Constant6 : Constant  Value=dt5
  Constant7 : Constant  Value=t_start5_2
  Constant9 : Constant  Value=t_start5_1
  Subsystem1 : Subsystem
  Subsystem3 : Subsystem
  tag scope: V_1=global, V_2=global
  wires:
  Subsystem3/1(P) -> [V_1]
  Constant30/1 -> Subsystem3/1(λ1)
  Constant31/1 -> Subsystem3/2(λ2)
  Constant33/1 -> Subsystem3/4(dP)
  Constant35/1 -> Subsystem3/6(dt)
  Constant34/1 -> Subsystem3/5(Pz)
  Constant32/1 -> Subsystem3/3(M)
  [trec2] -> Subsystem3/7(trec)
  Constant9/1 -> Subsystem3/8(t_start)
  Subsystem1/1(P) -> [V_2]
  Constant1/1 -> Subsystem1/1(λ1)
  Constant2/1 -> Subsystem1/2(λ2)
  Constant4/1 -> Subsystem1/4(dP)
  Constant6/1 -> Subsystem1/6(dt)
  Constant5/1 -> Subsystem1/5(Pz)
  Constant3/1 -> Subsystem1/3(M)
  [trec2] -> Subsystem1/7(trec)
  Constant7/1 -> Subsystem1/8(t_start)

== system station_no_recovery/Невосстанавливаемые объекты/Element Exponential ==
  note: интенсивность событий
      | в рассматриваемом потоке
  "lambda " : Inport
  Clock : Clock
  Divide : Product  Inputs=**
  Gain : Gain  Gain=-1
  Math Function : Math  SaturateOnIntegerOverflow=on
  P(t)1 : Outport
  wires:
  "lambda "/1 -> Divide/2
  Math Function/1 -> P(t)1/1
  Gain/1 -> Math Function/1
  Clock/1 -> Divide/1
  Divide/1 -> Gain/1

== system station_no_recovery/Невосстанавливаемые объекты/Element Exponential1 ==
  note: интенсивность событий
      | в рассматриваемом потоке
  "lambda " : Inport
  Clock : Clock
  Divide : Product  Inputs=**
  Gain : Gain  Gain=-1
  Math Function : Math  SaturateOnIntegerOverflow=on
  P(t)1 : Outport
  wires:
  Divide/1 -> Gain/1
  Clock/1 -> Divide/1
  Gain/1 -> Math Function/1
  Math Function/1 -> P(t)1/1
  "lambda "/1 -> Divide/2

== system station_no_recovery/Невосстанавливаемые объекты/Element Exponential2 ==
  note: интенсивность событий
      | в рассматриваемом потоке
  "lambda " : Inport
  Clock : Clock
  Divide : Product  Inputs=**
  Gain : Gain  Gain=-1
  Math Function : Math  SaturateOnIntegerOverflow=on
  P(t)1 : Outport
  wires:
  "lambda "/1 -> Divide/2
  Math Function/1 -> P(t)1/1
  Gain/1 -> Math Function/1
  Clock/1 -> Divide/1
  Divide/1 -> Gain/1

== system station_no_recovery/Невосстанавливаемые объекты/Element Exponential3 ==
  note: интенсивность событий
      | в рассматриваемом потоке
  "lambda " : Inport
  Clock : Clock
  Divide : Product  Inputs=**
  Gain : Gain  Gain=-1
  Math Function : Math  SaturateOnIntegerOverflow=on
  P(t)1 : Outport
  wires:
  Divide/1 -> Gain/1
  Clock/1 -> Divide/1
  Gain/1 -> Math Function/1
  Math Function/1 -> P(t)1/1
  "lambda "/1 -> Divide/2

== system station_no_recovery/Невосстанавливаемые объекты/Element Exponential4 ==
  note: интенсивность событий
      | в рассматриваемом потоке
  "lambda " : Inport
  Clock : Clock
  Divide : Product  Inputs=**
  Gain : Gain  Gain=-1
  Math Function : Math  SaturateOnIntegerOverflow=on
  P(t)1 : Outport
  wires:
  "lambda "/1 -> Divide/2
  Math Function/1 -> P(t)1/1
  Gain/1 -> Math Function/1
  Clock/1 -> Divide/1
  Divide/1 -> Gain/1

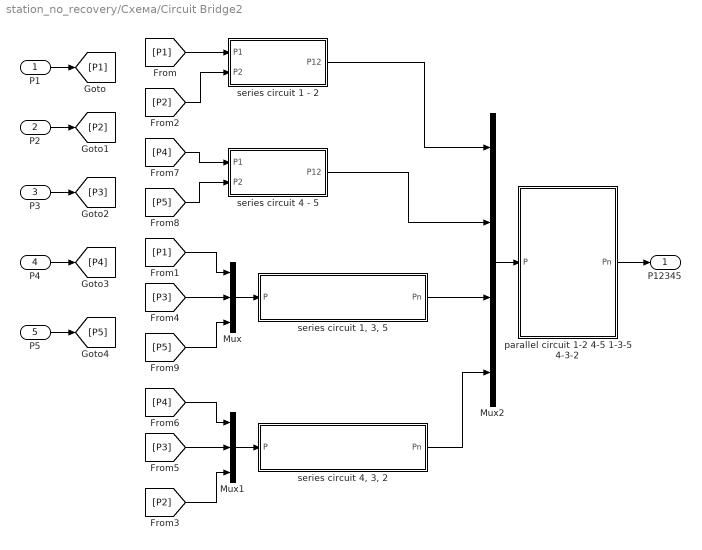
== system station_no_recovery/Схема/Сircuit Bridge2 ==
  P1 : Inport
  P2 : Inport  Port=2
  P3 : Inport  Port=3
  P4 : Inport  Port=4
  P5 : Inport  Port=5
  Mux : Mux  Inputs=3
  Mux1 : Mux  Inputs=3
  Mux2 : Mux
  parallel circuit 1-2 4-5 1-3-5 4-3-2 : Subsystem  mask(Сircuit n Parallel){}
      mask help:
      | <p>Возвращает вероятность безотказной работы n параллельно соединенных
      | элементов.</p>
      | <p>В системе с параллельной структурой отказ системы в целом происходит только
      | при отказе всех элементов.</p>
      mask Help:
      | <p>Возвращает вероятность безотказной работы n параллельно соединенных
      | элементов.</p>
      | <p>Входной параметр P - массив вероятностей безотказной работы элементов.</p>
      | <p>Выходной параметр Pт - вероятность безотказной работы n параллельно
      | соединенных элементов.</p>
      mask Display:
      | image('images\png\parallel.png')
      | port_label('input', 1, 'P')
      | port_label('output', 1, 'Pn')
  series circuit 1 - 2 : Subsystem  mask(Сircuit Series){}
      mask help:
      | <p>Возвращает вероятность безотказной работы двух последовательно соединенных
      | элементов.</p>
      | <p>В системе с последовательной структурой отказ любого компонента приводит
      | к отказу системы в целом.</p>
      mask Help:
      | <p>Возвращает вероятность безотказной работы двух последовательно соединенных
      | элементов.</p>
      | <p>Входные параметры:</p>
      | <p>P1 - вероятность безотказной работы первого элемента,</p>
      | <p>P2 - вероятность безотказной работы второго элемента.</p>
      | <p>Выходной параметр P12 - вероятность безотказной работы двух последовательно
      | соединенных элементов.</p>
      mask Display:
      | image('images/png/series2.png')
      | port_label('input', 1, 'P1')
      | port_label('input', 2, 'P2')
      | port_label('output', 1, 'P12')
  "series circuit 1, 3, 5" : Subsystem  mask(Сircuit n Series){}
      mask help:
      | <p>Возвращает вероятность безотказной работы n последовательно соединенных
      | элементов.</p>
      | <p>В системе с последовательной структурой отказ любого компонента приводит
      | к отказу системы в целом.</p>
      mask Help:
      | <p>Возвращает вероятность безотказной работы n последовательно соединенных
      | элементов.</p>
      | <p>Входной параметр P - массив вероятностей безотказной работы n элементов.</p>
      | <p>Выходной параметр Pn - вероятность безотказной работы n последовательно
      | соединенных элементов.</p>
      mask Display:
      | image('images\png\series.png')
      | port_label('input', 1, 'P')
      | port_label('output', 1, 'Pn')
  series circuit 4 - 5 : Subsystem  mask(Сircuit Series){}
      mask help:
      | <p>Возвращает вероятность безотказной работы двух последовательно соединенных
      | элементов.</p>
      | <p>В системе с последовательной структурой отказ любого компонента приводит
      | к отказу системы в целом.</p>
      mask Help:
      | <p>Возвращает вероятность безотказной работы двух последовательно соединенных
      | элементов.</p>
      | <p>Входные параметры:</p>
      | <p>P1 - вероятность безотказной работы первого элемента,</p>
      | <p>P2 - вероятность безотказной работы второго элемента.</p>
      | <p>Выходной параметр P12 - вероятность безотказной работы двух последовательно
      | соединенных элементов.</p>
      mask Display:
      | image('images/png/series2.png')
      | port_label('input', 1, 'P1')
      | port_label('input', 2, 'P2')
      | port_label('output', 1, 'P12')
  "series circuit 4, 3, 2" : Subsystem  mask(Сircuit n Series){}
      mask help:
      | <p>Возвращает вероятность безотказной работы n последовательно соединенных
      | элементов.</p>
      | <p>В системе с последовательной структурой отказ любого компонента приводит
      | к отказу системы в целом.</p>
      mask Help:
      | <p>Возвращает вероятность безотказной работы n последовательно соединенных
      | элементов.</p>
      | <p>Входной параметр P - массив вероятностей безотказной работы n элементов.</p>
      | <p>Выходной параметр Pn - вероятность безотказной работы n последовательно
      | соединенных элементов.</p>
      mask Display:
      | image('images\png\series.png')
      | port_label('input', 1, 'P')
      | port_label('output', 1, 'Pn')
  P12345 : Outport
  wires:
  P1/1 -> [P1]
  [P3] -> Mux1/2
  P5/1 -> [P5]
  [P5] -> Mux/3
  "series circuit 1, 3, 5"/1(Pn) -> Mux2/3
  [P4] -> Mux1/1
  [P3] -> Mux/2
  "series circuit 4, 3, 2"/1(Pn) -> Mux2/4
  P2/1 -> [P2]
  [P5] -> series circuit 4 - 5/2(P2)
  series circuit 1 - 2/1(P12) -> Mux2/1
  [P2] -> series circuit 1 - 2/2(P2)
  P3/1 -> [P3]
  series circuit 4 - 5/1(P12) -> Mux2/2
  parallel circuit 1-2 4-5 1-3-5 4-3-2/1(Pn) -> P12345/1
  [P1] -> Mux/1
  [P4] -> series circuit 4 - 5/1(P1)
  P4/1 -> [P4]
  [P1] -> series circuit 1 - 2/1(P1)
  Mux/1 -> "series circuit 1, 3, 5"/1(P)
  [P2] -> Mux1/3
  Mux1/1 -> "series circuit 4, 3, 2"/1(P)
  Mux2/1 -> parallel circuit 1-2 4-5 1-3-5 4-3-2/1(P)

== system station_no_recovery/Схема/Сircuit Parallel2 ==
  P1 : Inport
  P2 : Inport  Port=2
  Fcn1 : Fcn  Expr=1-((1-u(1))*(1-u(2)))
  Mux1 : Mux  Inputs=2
  P12 : Outport
  wires:
  P2/1 -> Mux1/2
  Mux1/1 -> Fcn1/1
  Fcn1/1 -> P12/1
  P1/1 -> Mux1/1

== system station_no_recovery/Схема/Сircuit Parallel3 ==
  P1 : Inport
  P2 : Inport  Port=2
  Fcn1 : Fcn  Expr=1-((1-u(1))*(1-u(2)))
  Mux1 : Mux  Inputs=2
  P12 : Outport
  wires:
  P1/1 -> Mux1/1
  Fcn1/1 -> P12/1
  Mux1/1 -> Fcn1/1
  P2/1 -> Mux1/2

== system station_no_recovery/Схема/Сircuit Series ==
  P1 : Inport
  P2 : Inport  Port=2
  Fcn : Fcn  Expr=u(1)*u(2)
  Mux : Mux  Inputs=2
  P12 : Outport
  wires:
  Mux/1 -> Fcn/1
  P1/1 -> Mux/1
  Fcn/1 -> P12/1
  P2/1 -> Mux/2

== system station_no_recovery/Схема/Сircuit Series1 ==
  P1 : Inport
  P2 : Inport  Port=2
  Fcn : Fcn  Expr=u(1)*u(2)
  Mux : Mux  Inputs=2
  P12 : Outport
  wires:
  P2/1 -> Mux/2
  Fcn/1 -> P12/1
  P1/1 -> Mux/1
  Mux/1 -> Fcn/1

== system station_no_recovery/Схема/Сircuit Series2 ==
  P1 : Inport
  P2 : Inport  Port=2
  Fcn : Fcn  Expr=u(1)*u(2)
  Mux : Mux  Inputs=2
  P12 : Outport
  wires:
  P2/1 -> Mux/2
  Fcn/1 -> P12/1
  P1/1 -> Mux/1
  Mux/1 -> Fcn/1

== system station_no_recovery/Схема/Сircuit Series3 ==
  P1 : Inport
  P2 : Inport  Port=2
  Fcn : Fcn  Expr=u(1)*u(2)
  Mux : Mux  Inputs=2
  P12 : Outport
  wires:
  Mux/1 -> Fcn/1
  P1/1 -> Mux/1
  Fcn/1 -> P12/1
  P2/1 -> Mux/2

== system station_no_recovery/Схема/Сircuit Series4 ==
  P1 : Inport
  P2 : Inport  Port=2
  Fcn : Fcn  Expr=u(1)*u(2)
  Mux : Mux  Inputs=2
  P12 : Outport
  wires:
  Mux/1 -> Fcn/1
  P1/1 -> Mux/1
  Fcn/1 -> P12/1
  P2/1 -> Mux/2

== system station_no_recovery/Схема/Сircuit n Parallel1 ==
  P : Inport
  n Parallel Function : MATLAB Function  TreatAsAtomicUnit=on
  Pn : Outport
  wires:
  P/1 -> n Parallel Function/1(P)
  n Parallel Function/1(Pn) -> Pn/1

== system station_no_recovery/Схема/Сircuit n Parallel2 ==
  P : Inport
  n Parallel Function : MATLAB Function  TreatAsAtomicUnit=on
  Pn : Outport
  wires:
  P/1 -> n Parallel Function/1(P)
  n Parallel Function/1(Pn) -> Pn/1

== system station_no_recovery/Схема/Сircuit n Parallel3 ==
  P : Inport
  n Parallel Function : MATLAB Function  TreatAsAtomicUnit=on
  Pn : Outport
  wires:
  n Parallel Function/1(Pn) -> Pn/1
  P/1 -> n Parallel Function/1(P)

== system station_no_recovery/Схема/Сircuit n Parallel4 ==
  P : Inport
  n Parallel Function : MATLAB Function  TreatAsAtomicUnit=on
  Pn : Outport
  wires:
  P/1 -> n Parallel Function/1(P)
  n Parallel Function/1(Pn) -> Pn/1

== system station_no_recovery/Схема/Сircuit n Parallel5 ==
  P : Inport
  n Parallel Function : MATLAB Function  TreatAsAtomicUnit=on
  Pn : Outport
  wires:
  n Parallel Function/1(Pn) -> Pn/1
  P/1 -> n Parallel Function/1(P)

== system station_no_recovery/Схема/Сircuit n Series5 ==
  P : Inport
  n Series Function : MATLAB Function  TreatAsAtomicUnit=on
  Pn : Outport
  wires:
  P/1 -> n Series Function/1(P)
  n Series Function/1(Pn) -> Pn/1

== system station_no_recovery/Схема/Сircuit n Series6 ==
  P : Inport
  n Series Function : MATLAB Function  TreatAsAtomicUnit=on
  Pn : Outport
  wires:
  n Series Function/1(Pn) -> Pn/1
  P/1 -> n Series Function/1(P)

== system station_no_recovery/Схема/Сircuit n Series7 ==
  P : Inport
  n Series Function : MATLAB Function  TreatAsAtomicUnit=on
  Pn : Outport
  wires:
  P/1 -> n Series Function/1(P)
  n Series Function/1(Pn) -> Pn/1

== system station_no_recovery/Схема/Сircuit n Series8 ==
  P : Inport
  n Series Function : MATLAB Function  TreatAsAtomicUnit=on
  Pn : Outport
  wires:
  n Series Function/1(Pn) -> Pn/1
  P/1 -> n Series Function/1(P)
